simulink library "Arithmetic_Operations_Lib"  (R2023a)
settings: Solver=ode45  StartTime=0.0  StopTime=10.0  RelTol=1e-3  EnableMultiTasking=on
libraries: Miscellaneous x202
(part 4 of 4)

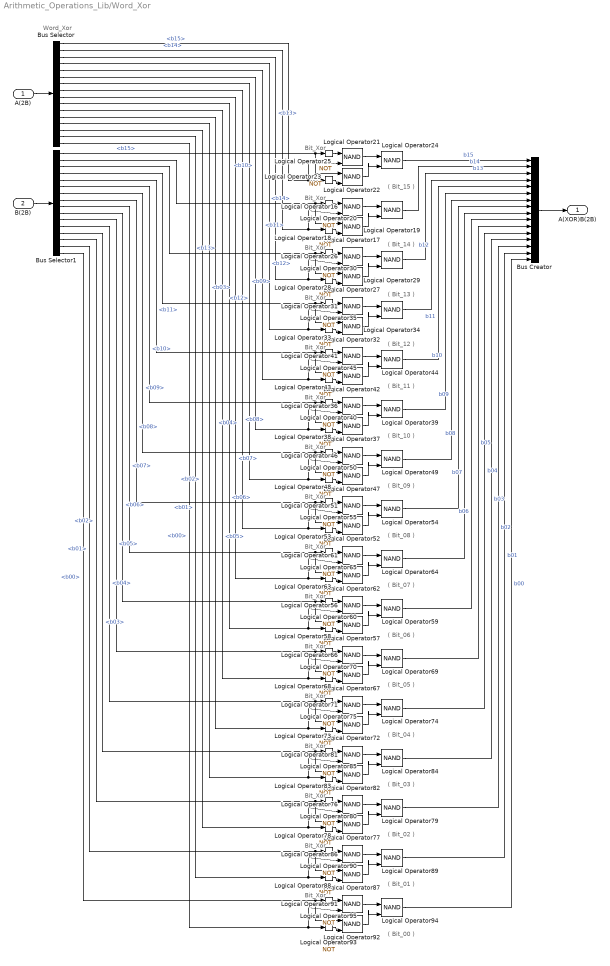
== system Arithmetic_Operations_Lib/Word_Xor ==
  note: Word_Xor
  note: Bit_Xor
  note: ( Bit_15 )
  note: ( Bit_14 )
  note: Bit_Xor
  note: ( Bit_13 )
  note: Bit_Xor
  note: ( Bit_12 )
  note: Bit_Xor
  note: ( Bit_08 )
  note: Bit_Xor
  note: ( Bit_10 )
  note: Bit_Xor
  note: Bit_Xor
  note: Bit_Xor
  note: ( Bit_11 )
  note: ( Bit_09 )
  note: Bit_Xor
  note: ( Bit_00 )
  note: ( Bit_01 )
  note: Bit_Xor
  note: ( Bit_02 )
  note: ( Bit_03 )
  note: Bit_Xor
  note: Bit_Xor
  note: ( Bit_04 )
  note: Bit_Xor
  note: ( Bit_06 )
  note: Bit_Xor
  note: Bit_Xor
  note: Bit_Xor
  note: ( Bit_07 )
  note: ( Bit_05 )
  A(2B) : Inport
  B(2B) : Inport  Port=2
  Bus Creator : BusCreator  Inputs=16
  Bus Selector : BusSelector  OutputSignals=b15,b14,b13,b12,b11,b10,b09,b08,b07,b06,b05,b04,b03,b02,b01,b00
  Bus Selector1 : BusSelector  OutputSignals=b15,b14,b13,b12,b11,b10,b09,b08,b07,b06,b05,b04,b03,b02,b01,b00
  Logical Operator{16..17,19,21..22,24,26..27,29,31..32,34,36..37,39,41..42,44,46..47,49,51..52,54,56..57,59,61..62,64,66..67,69,71..72,74,76..77,79,81..82,84,86..87,89,91..92,94} (48 alike) : Logic  Operator=NAND  IconShape=distinctive  AllPortsSameDT=off  OutDataTypeStr=boolean
  Logical Operator{18,20,23,25,28,30,33,35,38,40,43,45,48,50,53,55,58,60,63,65,68,70,73,75,78,80,83,85,88,90,93,95} (32 alike) : Logic  Operator=NOT  IconShape=distinctive  AllPortsSameDT=off  OutDataTypeStr=boolean
  A(XOR)B(2B) : Outport  OutputWhenDisabled=reset
  wires:
  Logical Operator23/1 -> Logical Operator22/2
  Bus Selector1/1 -> Logical Operator25/1, Logical Operator22/1  "<b15>"
  Logical Operator24/1 -> Bus Creator/1  "b15"
  Logical Operator22/1 -> Logical Operator24/2
  Logical Operator25/1 -> Logical Operator21/1
  Logical Operator21/1 -> Logical Operator24/1
  Logical Operator20/1 -> Logical Operator16/1
  Logical Operator16/1 -> Logical Operator19/1
  Logical Operator17/1 -> Logical Operator19/2
  Logical Operator18/1 -> Logical Operator17/2
  Logical Operator19/1 -> Bus Creator/2  "b14"
  Bus Selector1/2 -> Logical Operator20/1, Logical Operator17/1  "<b14>"
  Logical Operator30/1 -> Logical Operator26/1
  Logical Operator26/1 -> Logical Operator29/1
  Logical Operator27/1 -> Logical Operator29/2
  Logical Operator28/1 -> Logical Operator27/2
  Logical Operator29/1 -> Bus Creator/3  "b13"
  Bus Selector1/3 -> Logical Operator30/1, Logical Operator27/1  "<b13>"
  Logical Operator35/1 -> Logical Operator31/1
  Logical Operator31/1 -> Logical Operator34/1
  Logical Operator32/1 -> Logical Operator34/2
  Logical Operator33/1 -> Logical Operator32/2
  Logical Operator34/1 -> Bus Creator/4  "b12"
  Bus Selector1/4 -> Logical Operator35/1, Logical Operator32/1  "<b12>"
  Bus Selector/4 -> Logical Operator31/2, Logical Operator33/1  "<b12>"
  Logical Operator54/1 -> Bus Creator/8  "b08"
  Bus Selector1/8 -> Logical Operator55/1, Logical Operator52/1  "<b08>"
  Logical Operator51/1 -> Logical Operator54/1
  Logical Operator40/1 -> Logical Operator36/1
  Logical Operator53/1 -> Logical Operator52/2
  Bus Selector1/6 -> Logical Operator40/1, Logical Operator37/1  "<b10>"
  Bus Selector/6 -> Logical Operator36/2, Logical Operator38/1  "<b10>"
  Logical Operator37/1 -> Logical Operator39/2
  Logical Operator45/1 -> Logical Operator41/1
  Logical Operator52/1 -> Logical Operator54/2
  Logical Operator42/1 -> Logical Operator44/2
  Logical Operator36/1 -> Logical Operator39/1
  Logical Operator55/1 -> Logical Operator51/1
  Logical Operator44/1 -> Bus Creator/5  "b11"
  Bus Selector/8 -> Logical Operator51/2, Logical Operator53/1  "<b08>"
  Bus Selector1/5 -> Logical Operator45/1, Logical Operator42/1  "<b11>"
  Bus Selector/5 -> Logical Operator41/2, Logical Operator43/1  "<b11>"
  Logical Operator46/1 -> Logical Operator49/1
  Logical Operator41/1 -> Logical Operator44/1
  Logical Operator47/1 -> Logical Operator49/2
  Logical Operator39/1 -> Bus Creator/6  "b10"
  Logical Operator49/1 -> Bus Creator/7  "b09"
  Logical Operator48/1 -> Logical Operator47/2
  Logical Operator50/1 -> Logical Operator46/1
  Bus Selector1/7 -> Logical Operator50/1, Logical Operator47/1  "<b09>"
  Bus Selector/7 -> Logical Operator46/2, Logical Operator48/1  "<b09>"
  Logical Operator43/1 -> Logical Operator42/2
  Logical Operator38/1 -> Logical Operator37/2
  Logical Operator83/1 -> Logical Operator82/2
  Logical Operator78/1 -> Logical Operator77/2
  Logical Operator90/1 -> Logical Operator86/1
  Logical Operator88/1 -> Logical Operator87/2
  Logical Operator79/1 -> Bus Creator/14  "b02"
  Logical Operator89/1 -> Bus Creator/15  "b01"
  Bus Selector1/15 -> Logical Operator90/1, Logical Operator87/1  "<b01>"
  Logical Operator86/1 -> Logical Operator89/1
  Bus Selector/13 -> Logical Operator81/2, Logical Operator83/1  "<b03>"
  Bus Selector/15 -> Logical Operator86/2, Logical Operator88/1  "<b01>"
  Logical Operator87/1 -> Logical Operator89/2
  Logical Operator81/1 -> Logical Operator84/1
  Bus Selector1/13 -> Logical Operator85/1, Logical Operator82/1  "<b03>"
  Bus Selector/16 -> Logical Operator91/2, Logical Operator93/1  "<b00>"
  Logical Operator92/1 -> Logical Operator94/2
  Logical Operator76/1 -> Logical Operator79/1
  Logical Operator84/1 -> Bus Creator/13  "b03"
  Logical Operator85/1 -> Logical Operator81/1
  Logical Operator82/1 -> Logical Operator84/2
  Logical Operator95/1 -> Logical Operator91/1
  Logical Operator93/1 -> Logical Operator92/2
  Logical Operator77/1 -> Logical Operator79/2
  Bus Selector1/14 -> Logical Operator80/1, Logical Operator77/1  "<b02>"
  Logical Operator94/1 -> Bus Creator/16  "b00"
  Logical Operator74/1 -> Bus Creator/12  "b04"
  Bus Selector1/12 -> Logical Operator75/1, Logical Operator72/1  "<b04>"
  Logical Operator71/1 -> Logical Operator74/1
  Logical Operator60/1 -> Logical Operator56/1
  Logical Operator73/1 -> Logical Operator72/2
  Bus Selector1/10 -> Logical Operator60/1, Logical Operator57/1  "<b06>"
  Bus Selector/10 -> Logical Operator56/2, Logical Operator58/1  "<b06>"
  Logical Operator57/1 -> Logical Operator59/2
  Logical Operator65/1 -> Logical Operator61/1
  Logical Operator72/1 -> Logical Operator74/2
  Logical Operator62/1 -> Logical Operator64/2
  Logical Operator56/1 -> Logical Operator59/1
  Logical Operator75/1 -> Logical Operator71/1
  Logical Operator64/1 -> Bus Creator/9  "b07"
  Bus Selector/12 -> Logical Operator71/2, Logical Operator73/1  "<b04>"
  Bus Selector1/9 -> Logical Operator65/1, Logical Operator62/1  "<b07>"
  Bus Selector/9 -> Logical Operator61/2, Logical Operator63/1  "<b07>"
  Logical Operator80/1 -> Logical Operator76/1
  Logical Operator66/1 -> Logical Operator69/1
  Logical Operator61/1 -> Logical Operator64/1
  Logical Operator91/1 -> Logical Operator94/1
  Logical Operator67/1 -> Logical Operator69/2
  Logical Operator59/1 -> Bus Creator/10  "b06"
  Logical Operator69/1 -> Bus Creator/11  "b05"
  Logical Operator68/1 -> Logical Operator67/2
  Bus Selector/14 -> Logical Operator76/2, Logical Operator78/1  "<b02>"
  Logical Operator70/1 -> Logical Operator66/1
  Bus Selector1/11 -> Logical Operator70/1, Logical Operator67/1  "<b05>"
  Bus Selector/11 -> Logical Operator66/2, Logical Operator68/1  "<b05>"
  Logical Operator63/1 -> Logical Operator62/2
  Logical Operator58/1 -> Logical Operator57/2
  Bus Selector1/16 -> Logical Operator95/1, Logical Operator92/1  "<b00>"
  Bus Selector/1 -> Logical Operator21/2, Logical Operator23/1  "<b15>"
  Bus Selector/2 -> Logical Operator16/2, Logical Operator18/1  "<b14>"
  Bus Selector/3 -> Logical Operator26/2, Logical Operator28/1  "<b13>"
  Bus Creator/1 -> A(XOR)B(2B)/1
  B(2B)/1 -> Bus Selector1/1
  A(2B)/1 -> Bus Selector/1
